simulink model "model"  (R2025b)
settings: Solver=VariableStepAuto  StartTime=0.0  StopTime=20  RelTol=1e-3
libraries: matrix_library x4, slpidlib x1, uavutilslib x1
settings Model: PacingRate=112  Creator=achu  LastModifiedBy=achu

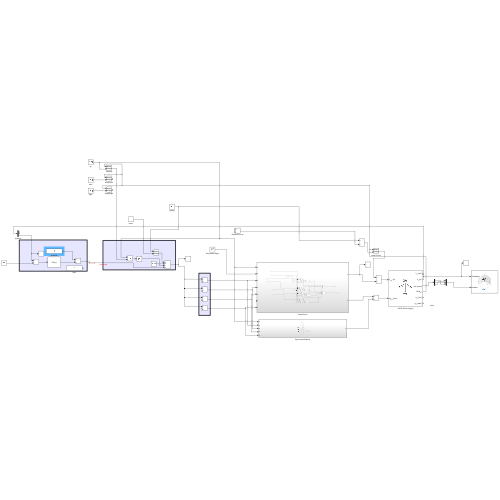
[thumbnail: Simulink's stored preview of the top-level diagram]
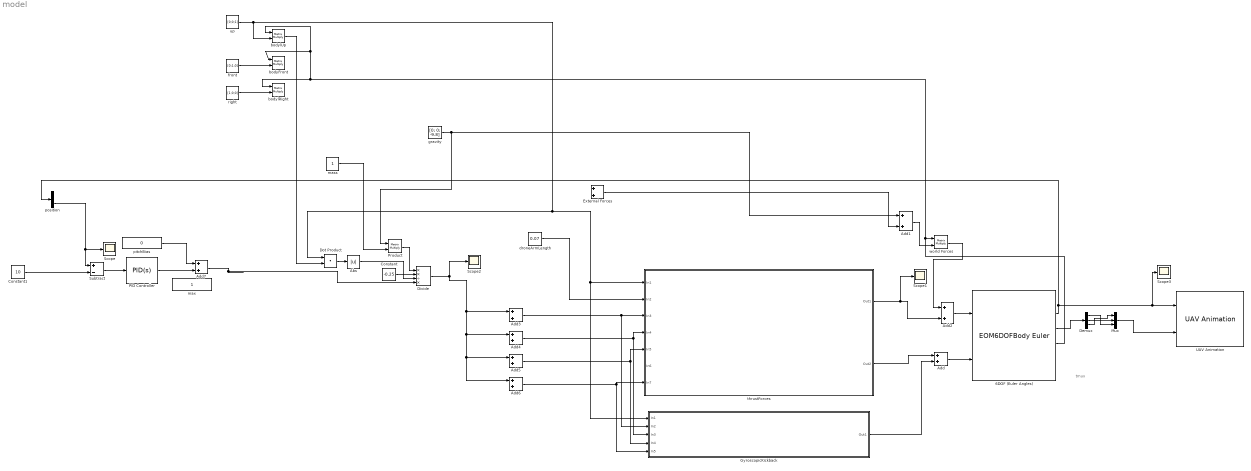
== system model ==
  note: tmux
  6DOF (Euler Angles) : EOM6DOFBodyEuler  eul_0=[0.02 0 0]
  Abs : Abs  SaturateOnIntegerOverflow=off
  Add{,1..7} (8 alike) : Sum
  Constant : Constant  Value=-0.25
  Constant1 : Constant  Value=10
  Demux : Demux  Outputs=3
  Divide : Product  Inputs=**/*
  Dot Product : DotProduct  OutDataTypeStr=Inherit: Inherit via internal rule
  External Forces : Sum
  GyroscopicKickback : Subsystem
  Mux : Mux  Inputs=3
  PID Controller : slpidlib/PID Controller  Controller=PID  Form=Parallel  TimeDomain=Continuous-time  UseExternalTs=off  SampleTime=-1  IntegratorMethod=Forward Euler  FilterMethod=Forward Euler  ControllerParametersSource=internal  P=-1  I=-0.2  UseKiTs=off  D=-0.8  UseExternalDerivativeSource=off  N=100  UseFilter=on  TunerSelectOption=Transfer Function Based (PID Tuner App)  InitialConditionSource=internal  InitialConditionForIntegrator=0  InitialConditionForFilter=0  DifferentiatorICPrevScaledInput=0  ExternalReset=none  TrackingMode=off  Kt=1  LimitOutput=off  SatLimitsSource=internal  UpperSaturationLimit=inf  LowerSaturationLimit=-inf  LinearizeAsGain=on  AntiWindupMode=none  Kb=1  LimitIntegrator=off  UpperIntegratorSaturationLimit=inf  LowerIntegratorSaturationLimit=-inf  POutMin=[]  POutMax=[]  IOutMin=[]  IOutMax=[]  DOutMin=[]  DOutMax=[]  NOutMin=[]  NOutMax=[]  SumOutMin=[]  SumOutMax=[]  SaturationOutMin=[]  SaturationOutMax=[]  PParamMin=[]  PParamMax=[]  IParamMin=[]  IParamMax=[]  DParamMin=[]  DParamMax=[]  NParamMin=[]  NParamMax=[]  KbParamMin=[]  KbParamMax=[]  KtParamMin=[]  KtParamMax=[]  KbOutMin=[]  KbOutMax=[]  KtOutMin=[]  KtOutMax=[]  IntegratorOutMin=[]  IntegratorOutMax=[]  FilterOutMin=[]  FilterOutMax=[]  SumI1OutMin=[]  SumI1OutMax=[]  SumI2OutMin=[]  SumI2OutMax=[]  SumI3OutMin=[]  SumI3OutMax=[]  SumI4OutMin=[]  SumI4OutMax=[]  SumDOutMin=[]  SumDOutMax=[]  DifferentiatorOutMin=[]  DifferentiatorOutMax=[]  FilterDiffOutCoefMin=[]  FilterDiffOutCoefMax=[]  ReciprocalOutMin=[]  ReciprocalOutMax=[]  SumDenOutMin=[]  SumDenOutMax=[]  SumNumOutMin=[]  SumNumOutMax=[]  DivideOutMin=[]  DivideOutMax=[]  UdiffTsProdOutMin=[]  UdiffTsProdOutMax=[]  NTsProdOutMin=[]  NTsProdOutMax=[]  UintegralTsProdOutMin=[]  UintegralTsProdOutMax=[]  UngainTsProdOutMin=[]  UngainTsProdOutMax=[]  ClampingZeroOutDataTypeStr=Inherit: Inherit via back propagation  ClampingZeroOutMin=[]  ClampingZeroOutMax=[]  FilterDenConstantOutDataTypeStr=Inherit: Inherit via back propagation  FilterDenConstantOutMin=[]  FilterDenConstantOutMax=[]  PCopyOutDataTypeStr=Inherit: Inherit via back propagation  PCopyOutMin=[]  PCopyOutMax=[]  NCopyOutDataTypeStr=Inherit: Inherit via back propagation  NCopyOutMin=[]  NCopyOutMax=[]  IntegratorContinuousStateAttributes=''  IntegratorStateMustResolveToSignalObject=off  IntegratorRTWStateStorageClass=Auto  FilterContinuousStateAttributes=''  FilterStateMustResolveToSignalObject=off  FilterRTWStateStorageClass=Auto  ParallelPVariant=InternalParameters  IdealPVariant=Disabled  IVariant=InternalParameters  DVariant=InternalParameters  IntegratorVariant=Continuous  SatVariant=Disabled  AWVariant=Passthrough  PCopyVariant=Disabled  TRVariant=Disabled  FdbkBlocksVariant=Forward  IdealPFdbkVariant=Disabled  SatFdbkVariant=Disabled  DerivativeFilterVariant=ContFilter  NVariant=InternalParameters  NCopyVariant=Disabled  FilterICVariant=InternalICsFilter  IntegratorICVariant=InternalICs  ExternalResetVariant=Disabled  TRSumVariant=Passthrough  SumFdbkVariant=Disabled  SumVariant=Sum_PID  TsampFilterVariant=InternalTs  TsampNgainVariant=Passthrough  TsampIntegralVariant=Disabled_SignalSpec  ExternalSaturationOutDataTypeStr=Inherit: Same as second input  DerivativeSourceVariant=ErrorSignal  PreIntVariant=InternalPreInt
  Product : Product  Multiplication=Matrix(*)
  Scope{,1..3} (4 alike) : Scope
      Scope settings: ActiveDisplayYMinimum=0.561749117999006  ActiveDisplayYMaximum=27.239136605292877
      Scope1 settings: ActiveDisplayYMinimum=-1  ActiveDisplayYMaximum=1
      Scope2 settings: ActiveDisplayYMinimum=-853.91857635505107  ActiveDisplayYMaximum=1291.7103665303814  DataLoggingVariableName=ScopeData2
      Scope3 settings: ActiveDisplayYMinimum=-146.66616230294065  ActiveDisplayYMaximum=489.22748668542886  DataLoggingVariableName=ScopeData3
  Subtract : Sum  Inputs=+-
  UAV Animation : uavutilslib/UAV Animation  NumUAV=1  DynamicUAVConfig=off  UAVType=Multirotor  UAVSize=1  UAVColor=[1 0 0]  UAVTrajectoryAlpha=1  InertialZDirection=Up  RotationFormat=Euler ZYX  DrawMarkers=off  SampleTime=-1
  bodyFront : Product  Multiplication=Matrix(*)
  bodylRight : Product  Multiplication=Matrix(*)
  bodylUp : Product  Multiplication=Matrix(*)
  droneArmLength : Constant  Value=0.07  VectorParams1D=off
  front : Constant  Value=[0;1;0]  VectorParams1D=off
  gravity : Constant  Value=[0; 0; -9.8]  VectorParams1D=off
  mass : Constant
  max : Constant
  pitchBias : Constant  Value=0
  position : Demux  Outputs=3
  right : Constant  Value=[1;0;0]  VectorParams1D=off
  thrustForces : Subsystem
  up : Constant  Value=[0;0;1]  VectorParams1D=off
  world Forces : Product  Multiplication=Matrix(*)
  wires:
  6DOF (Euler Angles)/2 -> Scope3/1, UAV Animation/1, position/1
  Add1/1 -> world Forces/2
  gravity/1 -> Add1/1, Product/1
  world Forces/1 -> Add2/1
  6DOF (Euler Angles)/4 -> bodylRight/1, bodyFront/1, bodylUp/1, world Forces/1
  Add2/1 -> 6DOF (Euler Angles)/1
  6DOF (Euler Angles)/3 -> Demux/1
  Demux/3 -> Mux/1
  Demux/2 -> Mux/2
  Demux/1 -> Mux/3
  Mux/1 -> UAV Animation/2
  External Forces/1 -> Add1/2
  droneArmLength/1 -> thrustForces/2(In2)
  Add5/1 -> thrustForces/5(In5), GyroscopicKickback/4(In4)
  thrustForces/1(Out1) -> Scope1/1, Add2/2
  thrustForces/2(Out2) -> Add/1
  Add/1 -> 6DOF (Euler Angles)/2
  Add3/1 -> GyroscopicKickback/2(In2), thrustForces/3(In3)
  Add4/1 -> thrustForces/4(In4), GyroscopicKickback/3(In3)
  Add6/1 -> thrustForces/7(In7), GyroscopicKickback/5(In5)
  GyroscopicKickback/1(Out1) -> Add/2
  bodylUp/1 -> Dot Product/2
  Dot Product/1 -> Abs/1
  Abs/1 -> Divide/3
  mass/1 -> Product/2
  Product/1 -> Divide/1
  Divide/1 -> Scope2/1, Add3/1, Add4/1, Add6/1, Add5/1
  Constant/1 -> Divide/2
  position/3 -> Scope/1, Subtract/1
  Subtract/1 -> PID Controller/1
  Constant1/1 -> Subtract/2
  Add7/1 -> Divide/4
  pitchBias/1 -> Add7/1
  PID Controller/1 -> Add7/2
  front/1 -> bodyFront/2
  right/1 -> bodylRight/2
  up/1 -> bodylUp/2, Dot Product/1, GyroscopicKickback/1(In1), thrustForces/1(In1)
  ? -> ?

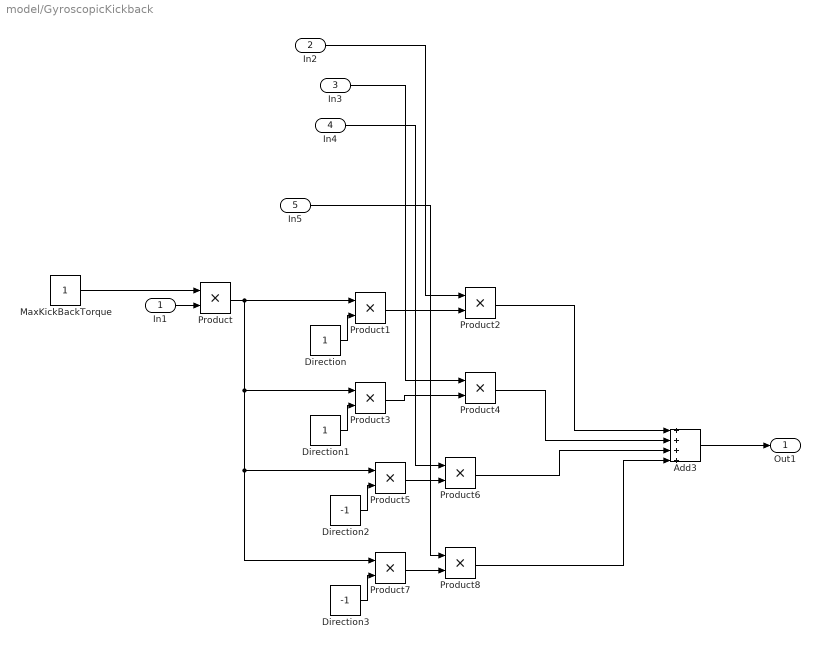
== system model/GyroscopicKickback ==
  In1 : Inport
  In2 : Inport  Port=2
  In3 : Inport  Port=3
  In4 : Inport  Port=4
  In5 : Inport  Port=5
  Add3 : Sum  Inputs=++++
  Direction : Constant
  Direction1 : Constant
  Direction2 : Constant  Value=-1
  Direction3 : Constant  Value=-1
  MaxKickBackTorque : Constant
  Product{,1..8} (9 alike) : Product
  Out1 : Outport
  wires:
  Product8/1 -> Add3/4
  In1/1 -> Product/2
  Product1/1 -> Product2/2
  Product3/1 -> Product4/2
  Product6/1 -> Add3/3
  MaxKickBackTorque/1 -> Product/1
  In2/1 -> Product2/1
  In4/1 -> Product6/1
  Product4/1 -> Add3/2
  Direction/1 -> Product1/2
  Direction2/1 -> Product5/2
  Add3/1 -> Out1/1
  Direction3/1 -> Product7/2
  Product/1 -> Product1/1, Product3/1, Product5/1, Product7/1
  Product5/1 -> Product6/2
  In3/1 -> Product4/1
  Product2/1 -> Add3/1
  Direction1/1 -> Product3/2
  In5/1 -> Product8/1
  Product7/1 -> Product8/2

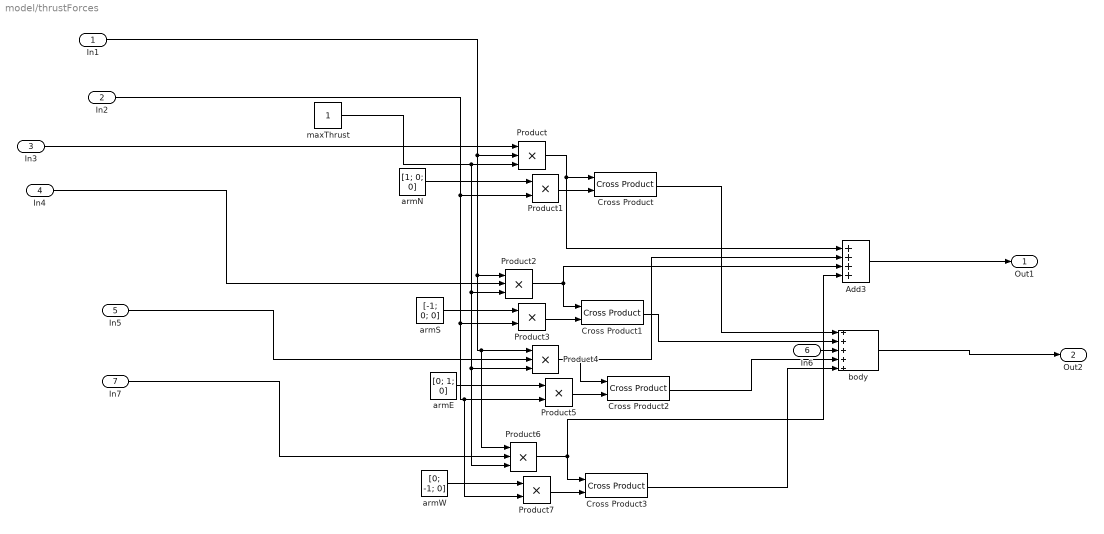
== system model/thrustForces ==
  In1 : Inport
  In2 : Inport  Port=2
  In3 : Inport  Port=3
  In4 : Inport  Port=4
  In5 : Inport  Port=5
  In6 : Inport  Port=6
  In7 : Inport  Port=7
  Add3 : Sum  Inputs=++++
  Cross Product{,1..3} (4 alike) : matrix_library/Cross Product
  Product{,2,4,6} (4 alike) : Product  Inputs=3
  Product{1,3,5,7} (4 alike) : Product
  armE : Constant  Value=[0; 1; 0]  VectorParams1D=off
  armN : Constant  Value=[1; 0; 0]  VectorParams1D=off
  armS : Constant  Value=[-1; 0; 0]  VectorParams1D=off
  armW : Constant  Value=[0; -1; 0]  VectorParams1D=off
  body : Sum  Inputs=+++++
  maxThrust : Constant
  Out1 : Outport
  Out2 : Outport  Port=2
  wires:
  armW/1 -> Product7/1
  Product1/1 -> Cross Product/2
  armS/1 -> Product3/1
  Cross Product/1 -> body/1
  Cross Product1/1 -> body/2
  Cross Product3/1 -> body/5
  Product/1 -> Cross Product/1, Add3/1
  In6/1 -> body/3
  In7/1 -> Product6/2
  body/1 -> Out2/1
  In5/1 -> Product4/2
  In4/1 -> Product2/2
  Cross Product2/1 -> body/4
  In1/1 -> Product4/1, Product6/1, Product2/1, Product/2
  In2/1 -> Product5/2, Product7/2, Product3/2, Product1/2
  armE/1 -> Product5/1
  Product3/1 -> Cross Product1/2
  armN/1 -> Product1/1
  Product2/1 -> Cross Product1/1, Add3/3
  In3/1 -> Product/1
  Product5/1 -> Cross Product2/2
  Product6/1 -> Add3/4, Cross Product3/1
  Product4/1 -> Add3/2, Cross Product2/1
  Product7/1 -> Cross Product3/2
  Add3/1 -> Out1/1
  maxThrust/1 -> Product4/3, Product6/3, Product2/3, Product/3
